simulink model "RRRsimulink"  (R2018b)
settings: Solver=VariableStepAuto  StartTime=0.0  StopTime=10.0  RelTol=1e-3
settings Model: Creator=Young Wang  LastModifiedBy=Young Wang

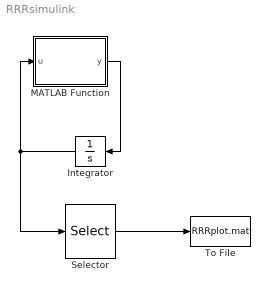
== system RRRsimulink ==
  Integrator : Integrator
  MATLAB Function : MATLAB Function  TreatAsAtomicUnit=on
  Selector : Selector  InputPortWidth=6  IndexOptions=Index vector (dialog)  Indices=[1 3 5]  OutputSizes=1
  To File : ToFile  Filename=RRRplot.mat  SaveFormat=Timeseries
  wires:
  MATLAB Function/1(y) -> Integrator/1
  Integrator/1 -> MATLAB Function/1(u), Selector/1
  Selector/1 -> To File/1

== matlab function RRRsimulink/MATLAB Function ==
  data: u input; y output
function y = fcn(u)

y = u;
